simulink model "sunsensor_processing_test"  (R2018b)
settings: Solver=FixedStepAuto  StartTime=0.0  StopTime=10.0  FixedStep=simParams.sample_time_s  RelTol=1e-3
libraries: simulink x2, sunsensor_processing_lib x1
settings Model: Creator=Taylor  LastModifiedBy=Taylor

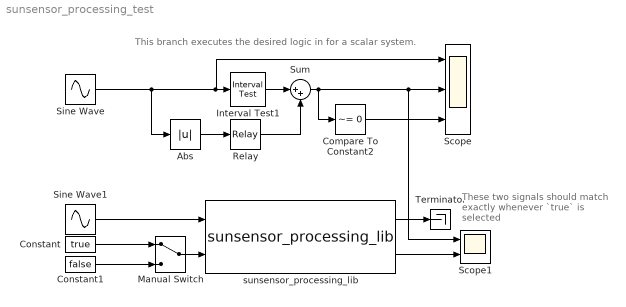
== system sunsensor_processing_test ==
  note: These two signals
      | should match exactly
      | whenever `true` is selected
  note: This branch executes the desired logic in for a scalar system.
  Abs : Abs
  Compare To Constant2 : simulink/Logic and Bit Operations/Compare To Constant  relop=~=  const=0  OutDataTypeStr=boolean
  Constant : Constant  Value=true
  Constant1 : Constant  Value=false
  Interval Test1 : simulink/Logic and Bit Operations/Interval Test  IntervalClosedRight=on  uplimit=60  IntervalClosedLeft=on  lowlimit=-60  OutDataTypeStr=uint8
  Manual Switch : ManualSwitch
  Relay : Relay  OnSwitchValue=60  OffSwitchValue=10  OnOutputValue=0  OffOutputValue=1
  Scope : Scope  NumInputPorts=3
  Scope1 : Scope  NumInputPorts=2
  Sine Wave : Sin  Amplitude=90  SampleTime=0
  Sine Wave1 : Sin  Amplitude=[90 90]  Bias=[0 0]  Frequency=[1 1]  Phase=[0 0]  SampleTime=0
  Sum : Sum  Inputs=|++
  Terminator : Terminator
  sunsensor_processing_lib : sunsensor_processing_lib/sunsensor_processing_lib  SystemSampleTime=-1
  wires:
  Relay/1 -> Sum/2
  Sum/1 -> Compare To Constant2/1, Scope/2, Scope1/1
  Sine Wave/1 -> Scope/1, Interval Test1/1, Abs/1
  Interval Test1/1 -> Sum/1
  Compare To Constant2/1 -> Scope/3
  Sine Wave1/1 -> sunsensor_processing_lib/1
  Manual Switch/1 -> sunsensor_processing_lib/2
  Constant1/1 -> Manual Switch/2
  Constant/1 -> Manual Switch/1
  sunsensor_processing_lib/1 -> Terminator/1
  sunsensor_processing_lib/2 -> Scope1/2
  Abs/1 -> Relay/1
